simulink model "DescreatIntegratorDiffer"  (Simulink 7.3)
settings: Solver=ode45  StartTime=0.0  StopTime=10  RelTol=1e-3
undefined symbols (not defined in the file or in its folder): DiscIntNeverNeededParam
libraries: simulink x1
settings Model: Creator=Sainquake Notebook  LastModifiedBy=Sainquake  BufferReuse=off
settings OptimizationCC: BlockReduction=off  InlineParams=on  BufferReuse=off
settings DebuggingCC: AlgebraicLoopMsg=none  SolverPrmCheckMsg=none  UnconnectedInputMsg=none  UnconnectedOutputMsg=none  UnconnectedLineMsg=none

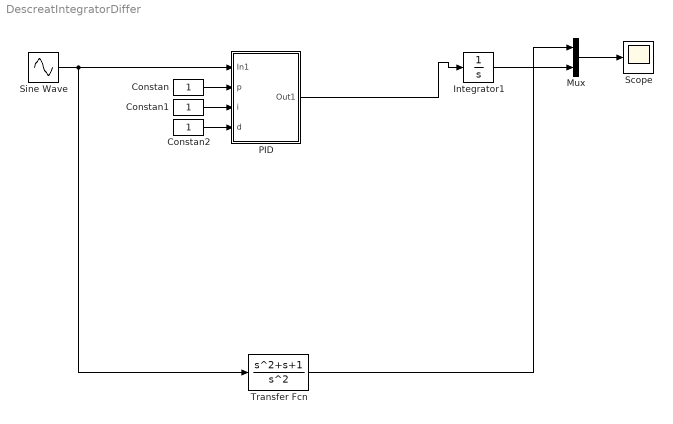
== system DescreatIntegratorDiffer ==
  Constan : Constant  OutDataType=fixdt(1, 16)  OutScaling=2^0
  Constan1 : Constant  OutDataType=fixdt(1, 16)  OutScaling=2^0
  Constan2 : Constant  OutDataType=fixdt(1, 16)  OutScaling=2^0
  Integrator1 : Integrator
  Mux : Mux  Inputs=2
  PID : Subsystem
  Scope : Scope
  Sine Wave : Sin  Amplitude=1  Bias=0  Frequency=1  Phase=0  Samples=10  SampleTime=0  Offset=0
  Transfer Fcn : TransferFcn  Numerator=[1 1 1]  Denominator=[1 0 0]
  wires:
  Sine Wave/1 -> PID/1(In1), Transfer Fcn/1
  Mux/1 -> Scope/1
  Integrator1/1 -> Mux/2
  Transfer Fcn/1 -> Mux/1
  PID/1(Out1) -> Integrator1/1
  Constan/1 -> PID/2(p)
  Constan1/1 -> PID/3(i)
  Constan2/1 -> PID/4(d)

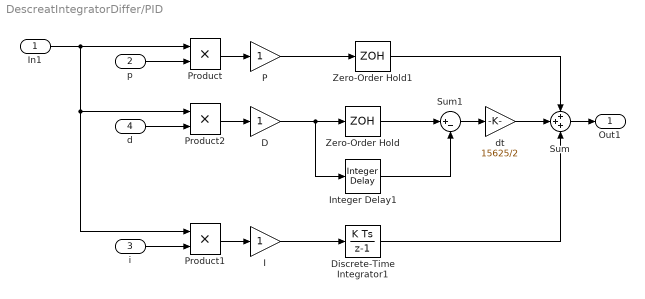
== system DescreatIntegratorDiffer/PID ==
  In1 : Inport  OutDataType=fixdt(1, 16)  OutScaling=2^0
  p : Inport  Port=2  OutDataType=fixdt(1, 16)  OutScaling=2^0
  i : Inport  Port=3  OutDataType=fixdt(1, 16)  OutScaling=2^0
  d : Inport  Port=4  OutDataType=fixdt(1, 16)  OutScaling=2^0
  D : Gain  ParameterDataType=fixdt(1, 16)  ParameterScaling=2^0  OutDataType=fixdt(1, 16)  OutScaling=2^0
  Discrete-Time Integrator1 : DiscreteIntegrator  SampleTime=2/15625  OutDataType=fixdt(1, 16)  OutScaling=2^0  ICPrevOutput=DiscIntNeverNeededParam  ICPrevScaledInput=DiscIntNeverNeededParam
  I : Gain  ParameterDataType=fixdt(1, 16)  ParameterScaling=2^0  OutDataType=fixdt(1, 16)  OutScaling=2^0
  Integer Delay1 : simulink/Discrete/Integer Delay  vinit=0.0  samptime=2/15625  NumDelays=1
  P : Gain  ParameterDataType=fixdt(1, 16)  ParameterScaling=2^0  OutDataType=fixdt(1, 16)  OutScaling=2^0
  Product : Product  OutDataType=fixdt(1, 16)  OutScaling=2^0  RndMeth=Zero
  Product1 : Product  OutDataType=fixdt(1, 16)  OutScaling=2^0  RndMeth=Zero
  Product2 : Product  OutDataType=fixdt(1, 16)  OutScaling=2^0  RndMeth=Zero
  Sum : Sum  Inputs=+++  OutDataType=fixdt(1, 16)  OutScaling=2^0
  Sum1 : Sum  Inputs=|+-  OutDataType=fixdt(1, 16)  OutScaling=2^0
  Zero-Order Hold : ZeroOrderHold  SampleTime=2/15625
  Zero-Order Hold1 : ZeroOrderHold  SampleTime=2/15625
  dt : Gain  Gain=15625/2  ParameterDataType=fixdt(1, 16)  ParameterScaling=2^0  OutDataType=fixdt(1, 16)  OutScaling=2^0
  Out1 : Outport  OutDataType=fixdt(1, 16)  OutScaling=2^0
  wires:
  Zero-Order Hold/1 -> Sum1/1
  Sum1/1 -> dt/1
  Integer Delay1/1 -> Sum1/2
  D/1 -> Integer Delay1/1, Zero-Order Hold/1
  dt/1 -> Sum/2
  Zero-Order Hold1/1 -> Sum/1
  P/1 -> Zero-Order Hold1/1
  I/1 -> Discrete-Time Integrator1/1
  Discrete-Time Integrator1/1 -> Sum/3
  Sum/1 -> Out1/1
  Product/1 -> P/1
  In1/1 -> Product/1, Product2/1, Product1/1
  p/1 -> Product/2
  Product2/1 -> D/1
  Product1/1 -> I/1
  d/1 -> Product2/2
  i/1 -> Product1/2
